simulink model "CartesianOrbitPropagator"  (R2023a)
settings: Solver=ode4  StartTime=0.0  StopTime=10.0  FixedStep=6000  RelTol=1e-3
settings Model: Creator=ndelurgio  LastModifiedBy=ndelurgio

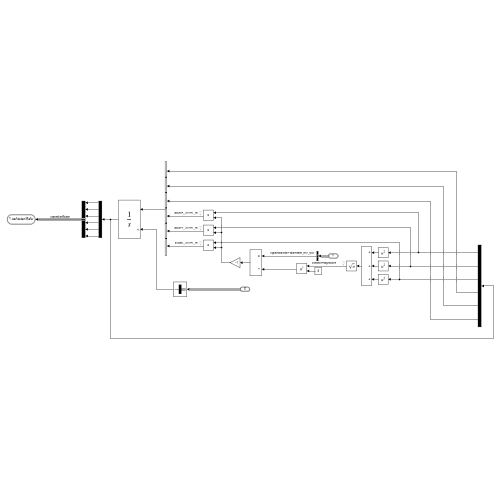
[thumbnail: Simulink's stored preview of the top-level diagram]
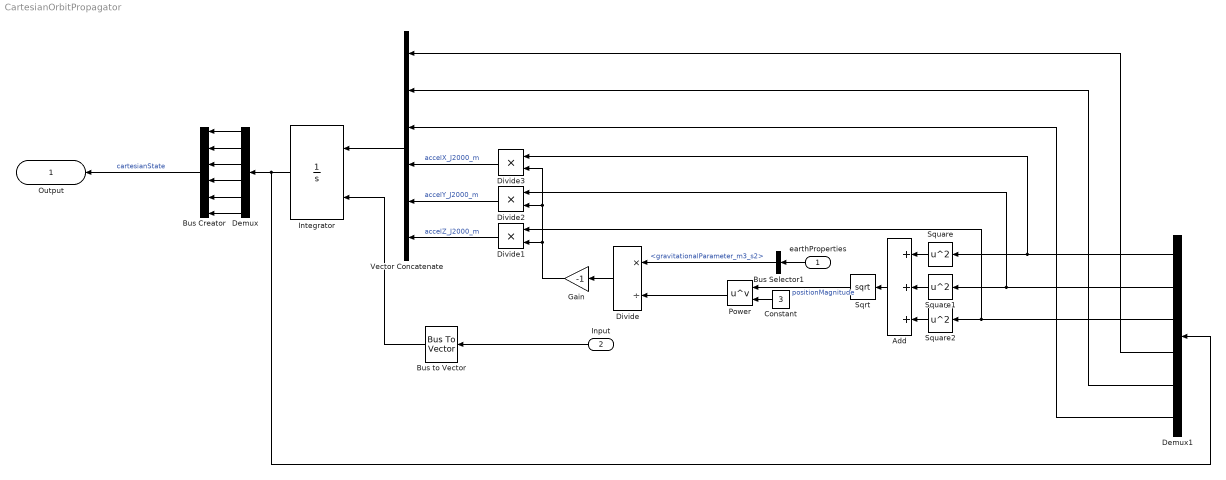
== system CartesianOrbitPropagator ==
  earthProperties : Inport  OutDataTypeStr=Bus: earthProperties
  Input : Inport  Port=2  OutDataTypeStr=Bus: cartesianState
  Add : Sum  Inputs=+++
  Bus Creator : BusCreator  Inputs=6  OutDataTypeStr=Bus: cartesianState  NonVirtualBus=on
      settings: InheritFromInputs=off
  Bus Selector1 : BusSelector  OutputSignals=gravitationalParameter_m3_s2
  Bus to Vector : BusToVector
  Constant : Constant  Value=3
  Demux : Demux  Outputs=6
  Demux1 : Demux  Outputs=6
  Divide : Product  Inputs=*/  OutDataTypeStr=double
  Divide1 : Product  Inputs=**
  Divide2 : Product  Inputs=**
  Divide3 : Product  Inputs=**
  Gain : Gain  Gain=-1  OutDataTypeStr=double
  Integrator : Integrator  InitialConditionSource=external
  Power : Math  Operator=pow
  Sqrt : Sqrt  OutDataTypeStr=double
  Square : Math  Operator=square
  Square1 : Math  Operator=square
  Square2 : Math  Operator=square
  Vector Concatenate : Concatenate  NumInputs=6
  Output : Outport  OutDataTypeStr=Bus: cartesianState
  wires:
  Bus Selector1/1 -> Divide/1  "<gravitationalParameter_m3_s2>"
  earthProperties/1 -> Bus Selector1/1
  Demux1/1 -> Divide3/1, Square/1
  Demux1/2 -> Divide2/1, Square1/1
  Demux1/3 -> Divide1/1, Square2/1
  Demux1/4 -> Vector Concatenate/1
  Demux1/5 -> Vector Concatenate/2
  Demux1/6 -> Vector Concatenate/3
  Square2/1 -> Add/3
  Square/1 -> Add/1
  Square1/1 -> Add/2
  Add/1 -> Sqrt/1
  Sqrt/1 -> Power/1  "positionMagnitude"
  Divide/1 -> Gain/1
  Gain/1 -> Divide3/2, Divide2/2, Divide1/2
  Divide3/1 -> Vector Concatenate/4  "accelX_J2000_m"
  Divide2/1 -> Vector Concatenate/5  "accelY_J2000_m"
  Divide1/1 -> Vector Concatenate/6  "accelZ_J2000_m"
  Vector Concatenate/1 -> Integrator/1
  Input/1 -> Bus to Vector/1
  Bus to Vector/1 -> Integrator/2
  Integrator/1 -> Demux1/1, Demux/1
  Demux/1 -> Bus Creator/1
  Demux/2 -> Bus Creator/2
  Demux/3 -> Bus Creator/3
  Demux/4 -> Bus Creator/4
  Demux/5 -> Bus Creator/5
  Demux/6 -> Bus Creator/6
  Bus Creator/1 -> Output/1  "cartesianState"
  Constant/1 -> Power/2
  Power/1 -> Divide/2
